simulink library "lib_InverterManager"  (R2017a)
settings: Solver=VariableStepAuto  StartTime=0.0  StopTime=10.0  RelTol=1e-3
libraries: simulink x1
settings Model: Creator=Di Russo  LastModifiedBy=Vraj M

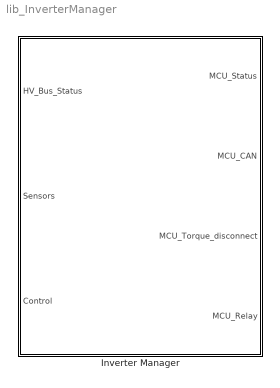
== system lib_InverterManager ==
  Inverter Manager : Subsystem

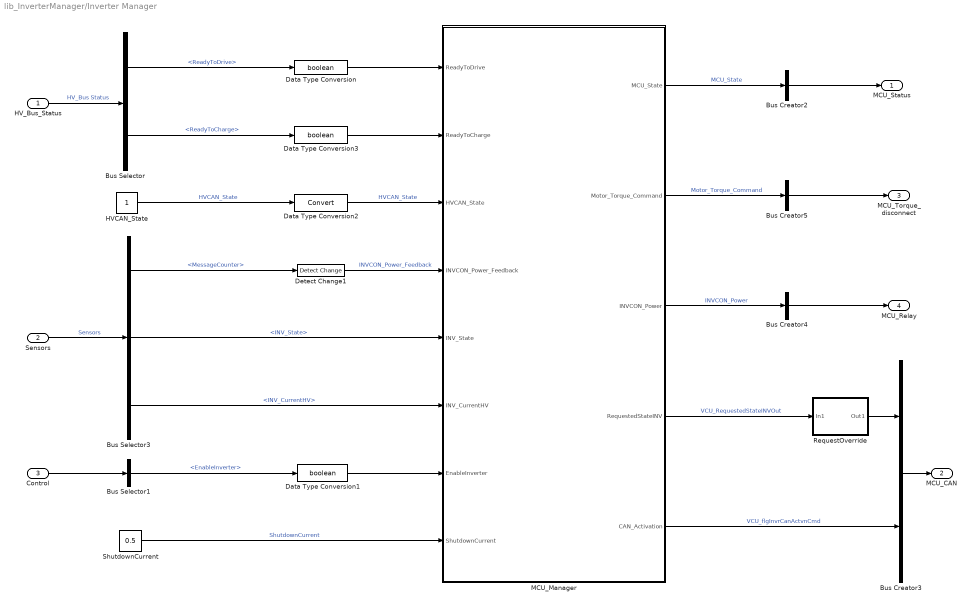
== system lib_InverterManager/Inverter Manager ==
  HV_Bus_Status : Inport
  Sensors : Inport  Port=2
  Control : Inport  Port=3
  Bus Creator2 : BusCreator  Inputs=1
  Bus Creator3 : BusCreator  Inputs=2
  Bus Creator4 : BusCreator  Inputs=1
  Bus Creator5 : BusCreator  Inputs=1
  Bus Selector : BusSelector  OutputSignals=ReadyToDrive,ReadyToCharge
  Bus Selector1 : BusSelector  OutputSignals=EnableInverter
  Bus Selector3 : BusSelector  OutputSignals=from_CAN.fromHV_CAN.from_MCU.INV_VCU_01.MessageCounter,from_CAN.fromHV_CAN.from_MCU.INV_VCU_01.INV_State,from_CAN.fromHV_CAN.from_MCU.INV_VCU_01.INV_CurrentHV
  Data Type Conversion : DataTypeConversion  OutDataTypeStr=boolean
  Data Type Conversion1 : DataTypeConversion  OutDataTypeStr=boolean
  Data Type Conversion2 : DataTypeConversion
  Data Type Conversion3 : DataTypeConversion  OutDataTypeStr=boolean
  Detect Change1 : simulink/Logic and Bit Operations/Detect Change  vinit=0  OutDataTypeStr=boolean
  HVCAN_State : Constant
  "MCU_Manager " : Stateflow chart  RequirementInfo={} %GIDa_1cd9daad_3829_4fdc_873a_baad14f0ce28  TreatAsAtomicUnit=on
  RequestOverride : Subsystem
  ShutdownCurrent : Constant  Value=0.5
  MCU_Status : Outport
  MCU_CAN : Outport  Port=2
  MCU_Torque_disconnect : Outport  Port=3
  MCU_Relay : Outport  Port=4
  wires:
  RequestOverride/1(Out1) -> Bus Creator3/1
  "MCU_Manager "/4(RequestedStateINV) -> RequestOverride/1(In1)  "VCU_RequestedStateINVOut"
  Control/1 -> Bus Selector1/1
  "MCU_Manager "/5(CAN_Activation) -> Bus Creator3/2  "VCU_flgInvrCanActvnCmd"
  Detect Change1/1 -> "MCU_Manager "/4(INVCON_Power_Feedback)  "INVCON_Power_Feedback"
  Data Type Conversion3/1 -> "MCU_Manager "/2(ReadyToCharge)
  Bus Selector/2 -> Data Type Conversion3/1  "<ReadyToCharge>"
  Data Type Conversion2/1 -> "MCU_Manager "/3(HVCAN_State)  "HVCAN_State"
  Bus Creator3/1 -> MCU_CAN/1
  Sensors/1 -> Bus Selector3/1  "Sensors"
  Bus Selector1/1 -> Data Type Conversion1/1  "<EnableInverter>"
  HV_Bus_Status/1 -> Bus Selector/1  "HV_Bus Status"
  Bus Selector/1 -> Data Type Conversion/1  "<ReadyToDrive>"
  ShutdownCurrent/1 -> "MCU_Manager "/8(ShutdownCurrent)  "ShutdownCurrent"
  Bus Selector3/3 -> "MCU_Manager "/6(INV_CurrentHV)  "<INV_CurrentHV>"
  "MCU_Manager "/1(MCU_State) -> Bus Creator2/1  "MCU_State"
  Bus Creator2/1 -> MCU_Status/1
  "MCU_Manager "/3(INVCON_Power) -> Bus Creator4/1  "INVCON_Power"
  Bus Creator4/1 -> MCU_Relay/1
  "MCU_Manager "/2(Motor_Torque_Command) -> Bus Creator5/1  "Motor_Torque_Command"
  Bus Creator5/1 -> MCU_Torque_disconnect/1
  Data Type Conversion/1 -> "MCU_Manager "/1(ReadyToDrive)
  Data Type Conversion1/1 -> "MCU_Manager "/7(EnableInverter)
  Bus Selector3/2 -> "MCU_Manager "/5(INV_State)  "<INV_State>"
  Bus Selector3/1 -> Detect Change1/1  "<MessageCounter>"
  HVCAN_State/1 -> Data Type Conversion2/1  "HVCAN_State"

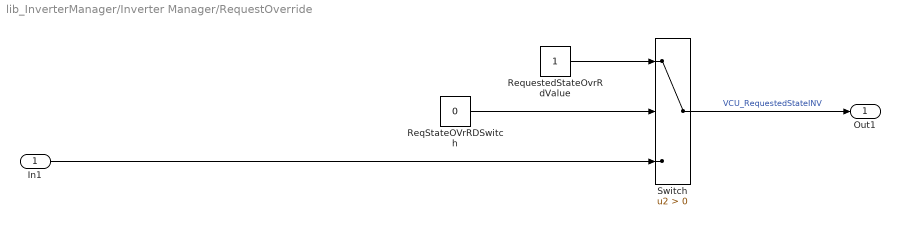
== system lib_InverterManager/Inverter Manager/RequestOverride ==
  In1 : Inport
  ReqStateOVrRDSwitch : Constant  Value=0
  RequestedStateOvrRdValue : Constant
  Switch : Switch  Criteria=u2 > Threshold
  Out1 : Outport
  wires:
  RequestedStateOvrRdValue/1 -> Switch/1
  ReqStateOVrRDSwitch/1 -> Switch/2
  In1/1 -> Switch/3
  Switch/1 -> Out1/1  "VCU_RequestedStateINV"

== stateflow chart lib_InverterManager/Inverter Manager/MCU_Manager  ==
  state MCU_Initialization
    state MCU_Request_Standby
      en:
      MCU_State = 1;
      RequestedStateINV = 3;
      CAN_Activation = 1;
    state Power_Off_INVCON
      entry:
      MCU_State = 0;
      INVCON_Power =0;
    state Power_On_INVCON
      en:MCU_State = 2;
      INVCON_Power =1;
    state HV_CAN_Actuation_Fault
      en:
      MCU_State = -1;
      CAN_Activation = 0;
    state INVCON_Power_Fault
      en:
      MCU_State = -2;
      INVCON_Power =0;
      CAN_Activation = 0;
    Power_Off_INVCON -> (junction 18) : {Timer=0;}
    (junction 18) -> MCU_Request_Standby [order 1] : [HVCAN_State]
    (default) -> Power_Off_INVCON
    HV_CAN_Actuation_Fault -> (junction 18) : [HVCAN_State]
    (junction 18) -> HV_CAN_Actuation_Fault [order 2] : after(3,sec)
    INVCON_Power_Fault -> (junction 18) : [~INVCON_Power_Feedback]
    MCU_Request_Standby -> Power_On_INVCON : after(5,sec)
    Power_On_INVCON -> INVCON_Power_Fault : after(5,sec)
        | [INV_State ~= 3]
  state MCU_ChargeMode
    state MCU_Ready
      en:
      MCU_State = 7;
    state MCU_Off
      en:
      MCU_State = 8;
      RequestedStateINV = 3;
    (default) -> MCU_ChargeMode.MCU_Ready
    MCU_ChargeMode.MCU_Ready -> MCU_ChargeMode.MCU_Off : [~ReadyToCharge]
  state MCU_TorqueMode
    state MCU_Enable
      en:MCU_State = 4;
      RequestedStateINV = 8;
      during: Timer = Timer + 1;
    state MCU_Ready
      en:
      MCU_State = 3;
    state MCU_Running
      en:
      MCU_State =5;
    state TorqueCommand_Reject_Fault
      en:
      MCU_State = -3;
    state MCU_Stop
      en:
      MCU_State = 6;
      RequestedStateINV = 3;
    (default) -> MCU_TorqueMode.MCU_Ready
    MCU_Enable -> (junction 35)
    (junction 35) -> MCU_Running [order 1] : [INV_State == 8]
    MCU_TorqueMode.MCU_Ready -> MCU_Enable : [EnableInverter]
        | {Timer = 0;}
    (junction 35) -> TorqueCommand_Reject_Fault [order 2] : after(5,sec)
    MCU_Running -> MCU_Stop : [~ReadyToDrive]
  state MCU_Shutdown
    state MCU_Off
      en:
      MCU_State = 10;
      RequestedStateINV = 0;
      during: Timer=Timer+1;
    state MCU_RdyForShtDwn
      en:
      MCU_State = 9;
    state MCU_Shtdwn_Cmplt
      en:
      MCU_State = 11;
      INVCON_Power =0;
      CAN_Activation = 0;
    state Motor_Isolate
      en:
      MCU_State = -5;
      INVCON_Power = 0;
      Motor_Torque_Command = 0;
    state ShutdownReq_Reject_Fault
      en:
      MCU_State = -4;
    (default) -> MCU_RdyForShtDwn
    MCU_RdyForShtDwn -> MCU_Shutdown.MCU_Off : [~EnableInverter]
        | {Timer = 0;}
    MCU_Shutdown.MCU_Off -> (junction 55)
    (junction 55) -> MCU_Shtdwn_Cmplt [order 2] : [INV_State == 0]
    (junction 55) -> ShutdownReq_Reject_Fault [order 1] : after(5,sec)
        | [INV_State == 14]
    ShutdownReq_Reject_Fault -> Motor_Isolate : after(3,sec)
  (default) -> MCU_Initialization
  MCU_Shutdown -> MCU_Initialization : [EnableInverter]
  MCU_TorqueMode -> MCU_Initialization [order 1] : [INV_State == 14]
  MCU_Initialization -> MCU_TorqueMode [order 2] : [INV_State == 3 &&...
      |  INVCON_Power_Feedback && ReadyToDrive]
  MCU_Initialization -> MCU_ChargeMode [order 1] : [INV_State == 3 &&...
      |  INVCON_Power_Feedback && ReadyToCharge]
  MCU_ChargeMode -> MCU_Initialization [order 2] : [INV_State == 14]
  MCU_TorqueMode -> MCU_Shutdown [order 2] : [INV_State == 3 && ~ReadyToDrive]
  MCU_ChargeMode -> MCU_Shutdown [order 1] : [INV_State == 3 && ~ReadyToCharge]
  data: ReadyToDrive input boolean; ReadyToCharge input; HVCAN_State input boolean; INVCON_Power_Feedback input; INV_State input; INV_CurrentHV input; Timer local double; MCU_State output; EnableInverter input boolean; ShutdownCurrent input; Motor_Torque_Command output; INVCON_Power output double; RequestedStateINV output; CAN_Activation output
